simulink model "TurtlebotOpenLoop"  (R2023b)
settings: Solver=VariableStepAuto  StartTime=0.0  StopTime=50  MaxStep=.1  RelTol=1e-3
undefined symbols (not defined in the file): q0, v_, w_
libraries: robotmobilelib x1
settings Model: Creator=tpoggi  LastModifiedBy=tpoggi

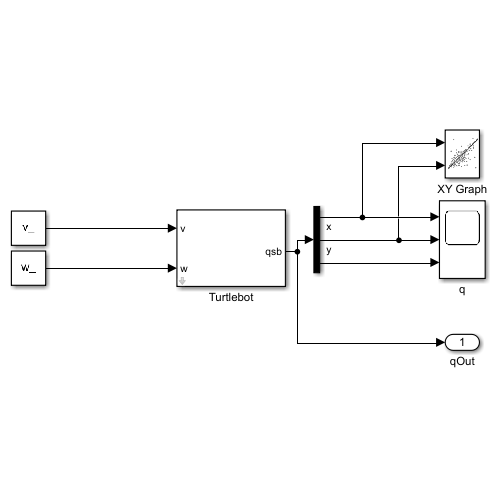
[thumbnail: Simulink's stored preview of the top-level diagram]
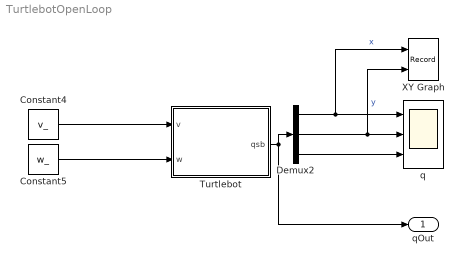
== system TurtlebotOpenLoop ==
  Constant4 : Constant  Value=v_
  Constant5 : Constant  Value=w_
  Demux2 : Demux  Outputs=3
  Turtlebot : Subsystem  mask{InitialState=q0}
      mask prompts: InitialState "robotics:robotslmobile:sharedblockmask:InitialStatePrompt"
      mask help:
      | Simple model of a turtlebot.
      |
      | Inputs:
      | - v: Linear velocity [m/s]
      | - w: Angular velocity [rad/s]
      |
      | Outputs:
      | - q: Configuration vector [x,y,phi]
      mask TypeOptions InitialState: Differential Drive Kinematic Model/InitialState
      mask DialogControl DescGroupVar Prompt: Description
      mask DialogControl ParameterGroupVar Prompt: Parameters:
      mask DialogControl InitialState Prompt: Initial state:
  XY Graph : Record  FileSettingsInternal="{\"entries\":[{\"content\":{\"excelSettings\":{\"content\":{},\"type\":\"Streamout.ExcelSettings\"}},\"type\":\"Streamout.FileSettingStorage\",\"uuid\":\"\"}],\"packageUris\":[\"http:\\/\\/schema.mathworks.com\\/mf0\\/streamout_blocks\\/R2020a\"],\"version\":\"1.0\"}"  Layout=[1 1]  SignalsInternal="{\"entries\":[{\"content\":{\"signals\":[{\"content\":{\"blockPath\":[],\"dimensions\":[1],\"domain\":\"\",\"lineColor\":\"#0072bd\",\"plots\":[ 1 ],\"port\":1,\"sid\":[\"\"],\"signalID\":1,\"signalName\":\"x\"},\"type\":\"RecordBlkView.Signal\",\"uuid\":\"\"},{\"content\":{\"blockPath\":[],\"dimensions\":[1],\"domain\":\"\",\"lineColor\":\"#d95319\",\"plots\":[ 1 ],\"port\":2,\"sid\":[\"\"],\"signalID\":2,\"signalName\":\"y\"},\"type\":\"RecordBlkView.Signal\",\"uuid\":\"\"}]},\"type\":\"RecordBlkView.InputSignals\",\"uuid\":\"\"}],\"packageUris\":[\"http:\\/\\/schema.mathworks.com\\/mf0\\/streamout_blocks\\/R2020a\"],\"version\":\"1.0\"}"  VisualizationBindings="{\"xyplotplugin\":{\"info\":[{\"series\":[{\"bindingParametersList\":[{\"parameter\":\"X-Axis\",\"signalID\":1,\"signalName\":\"x\"},{\"parameter\":\"Y-Axis\",\"signalID\":2,\"signalName\":\"y\"}],\"seriesID\":0}],\"subplotID\":1}]}}"  CompatibilityTag=XY
  q : Scope  NumInputPorts=3
  qOut : Outport
  wires:
  Constant5/1 -> Turtlebot/2(w)
  Demux2/1 -> q/1, XY Graph/1  "x"
  Demux2/2 -> q/2, XY Graph/2  "y"
  Constant4/1 -> Turtlebot/1(v)
  Turtlebot/1(qsb) -> qOut/1, Demux2/1
  Demux2/3 -> q/3

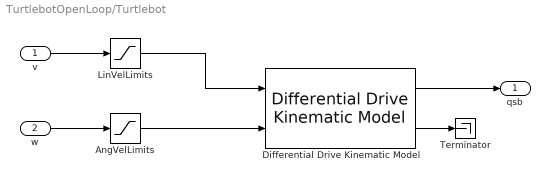
== system TurtlebotOpenLoop/Turtlebot ==
  v : Inport
  w : Inport  Port=2
  AngVelLimits : Saturate  UpperLimit=2.84  LowerLimit=-2.84
  Differential Drive Kinematic Model : robotmobilelib/Differential Drive Kinematic Model  VehicleInputs=Vehicle Speed & Heading Angular Velocity  WheelRadius=0.066  WheelSpeedRange=[-inf inf]  TrackWidth=0.16  InitialState=InitialState  SimulateUsing=Interpreted execution
  LinVelLimits : Saturate  UpperLimit=0.22  LowerLimit=-0.22
  Terminator : Terminator
  qsb : Outport
  wires:
  Differential Drive Kinematic Model/1 -> qsb/1
  v/1 -> LinVelLimits/1
  w/1 -> AngVelLimits/1
  Differential Drive Kinematic Model/2 -> Terminator/1
  LinVelLimits/1 -> Differential Drive Kinematic Model/1
  AngVelLimits/1 -> Differential Drive Kinematic Model/2
